simulink model "Fuzzy_Logic_MPPT_for_SolarPV"  (R2023b)
settings: Solver=ode45  StartTime=0.0  StopTime=10  RelTol=1e-3  EnableMultiTasking=on
PostLoadFcn:
  | fuzzyLogicDesigner('mppt')
libraries: spsSeriesRLCBranchLib x4, spsDiodeLib x2, fuzblock x1, spsPWMGeneratorDCDCLib x1, spsMosfetLib x1, spsPVArrayLib x1, spsVoltageMeasurementLib x1, sps_lib x1
settings Model: Creator=Niaz  LastModifiedBy=SUCHINTH
settings SolverCC: AlgebraicLoopSolver=TrustRegion
settings DataIOCC: LimitDataPoints=on  SaveFormat=Array  ReturnWorkspaceOutputs=off
settings OptimizationCC: LifeSpan=inf
settings DebuggingCC: UnconnectedInputMsg=warning  UnconnectedOutputMsg=warning  UnconnectedLineMsg=warning  SFUnexpectedBacktrackingDiag=warning  SFNoUnconditionalDefaultTransitionDiag=warning  SFExecutionAtInitializationDiag=none  ArithmeticOperatorsInVariantConditions=warning
settings HardwareCC: ProdBitPerPointer=32  ProdBitPerSizeT=32  ProdBitPerPtrDiffT=32  ProdLargestAtomicFloat=None  ProdIntDivRoundTo=Undefined  ProdEndianess=Unspecified  ProdWordSize=32  ProdHWDeviceType=32-bit Generic
settings ModelReferenceCC: EnableRefExpFcnMdlSchedulingChecks=on  PropagateSignalLabelsOutOfModel=off
settings SFSimCC: SimUseLocalCustomCode=off  CustomCodeUndefinedFunction=UseInterfaceOnly
settings RTWCC: RTWUseLocalCustomCode=off
settings CodeAppCC: StateflowObjectComments=on
settings GRTTargetCC: TargetLangStandard=C89/C90 (ANSI)
settings ConfigComp: CovMetricSettings=dw  CovSaveCumulativeToWorkspaceVar=on  CovSaveSingleToWorkspaceVar=on  CovExternalEMLEnable=off
settings SimscapeCC: SimscapeNormalizeSystem=off  SimscapeLogType=all  SimscapeLogSimulationStatistics=on  SimscapeLogOpenViewer=on

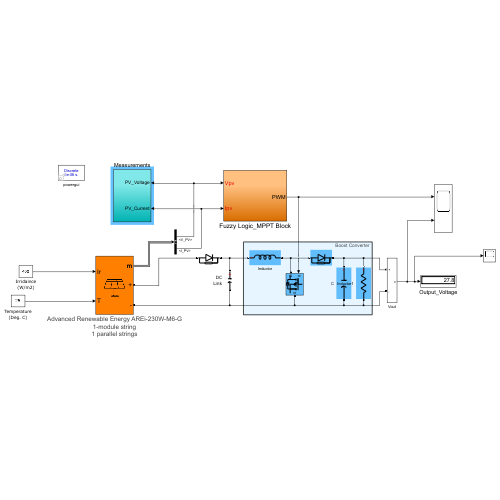
[thumbnail: Simulink's stored preview of the top-level diagram]
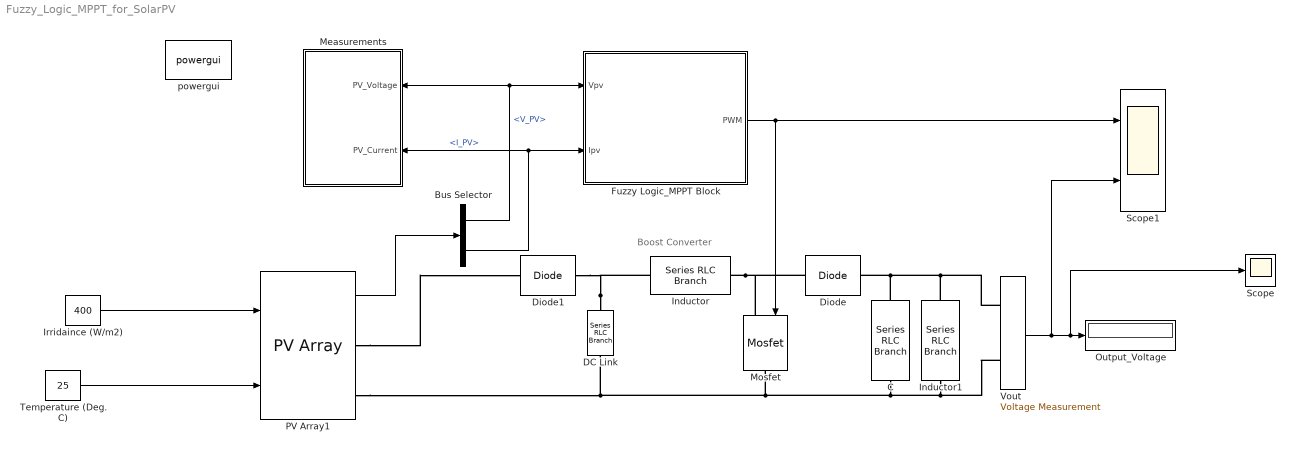
== system Fuzzy_Logic_MPPT_for_SolarPV ==
  note: Boost Converter
  Bus Selector : BusSelector  OutputSignals=V_PV,I_PV
  C : spsSeriesRLCBranchLib/Series RLC Branch  LConnTagsString=__new0  RConnTagsString=__new0  BranchType=C  Resistance=1  Inductance=1e-3  SetiL0=off  InitialCurrent=0  Capacitance=5000e-6  Setx0=off  InitialVoltage=600  Measurements=None
  DC Link : spsSeriesRLCBranchLib/Series RLC Branch  LConnTagsString=__new0  RConnTagsString=__new0  BranchType=C  Resistance=0.001  Inductance=1.0  SetiL0=off  InitialCurrent=0  Capacitance=4000e-6  Setx0=off  InitialVoltage=310  Measurements=None
  Diode : spsDiodeLib/Diode  Ron=0.001  Lon=0  Vf=0.8  IC=0  UseSnubber=off  Rs=500  Cs=250e-9  Measurements=off
  Diode1 : spsDiodeLib/Diode  Ron=0.001  Lon=0  Vf=0.8  IC=0  UseSnubber=off  Rs=500  Cs=250e-9  Measurements=off
  Fuzzy Logic_MPPT Block : Subsystem
  Inductor : spsSeriesRLCBranchLib/Series RLC Branch  LConnTagsString=__new0  RConnTagsString=__new0  BranchType=L  Resistance=0.01  Inductance=4e-4  SetiL0=off  InitialCurrent=5  Capacitance=1e-6  Setx0=off  InitialVoltage=0  Measurements=None
  Inductor1 : spsSeriesRLCBranchLib/Series RLC Branch  LConnTagsString=__new0  RConnTagsString=__new0  BranchType=R  Resistance=10  Inductance=4e-4  SetiL0=off  InitialCurrent=5  Capacitance=1e-6  Setx0=off  InitialVoltage=0  Measurements=None
  Irridaince (W/m2) : Constant  Value=400
  Measurements : Subsystem
  Mosfet : spsMosfetLib/Mosfet  Ron=0.1  Lon=0  Rd=0.01  Vfd=0  IC=0  Rs=1e5  Cs=inf  Measurements=off
  Output_Voltage : Display
  PV Array1 : spsPVArrayLib/PV Array  Npar=1  Nser=1  PlotType=one module @ 25 deg.C & specified irradiances  S_vec=[1000 800 400 200 100]  Temp_C_vec=[ 50 ]  ModuleName=Advanced Renewable Energy AREi-230W-M6-G  PlotWhenSelected=off  Pm=230.4  Ncell=60  Voc=37.14  Isc=8  Vm=30.72  Im=7.5  beta_Voc_pc=-0.35335  alpha_Isc_pc=0.05535  beta_Voc=-0.13123  alpha_Isc=0.004428  IL=8.007  I0=2.1265e-10  nI=0.99005  Rsh=280.3446  Rs=0.2449  RobustModel=off  RobustCellTemperature=313.3991  BAL=on  Tc=1e-6  Tfilter=5e-5
      settings: AttributesFormatString=|
      | %<ModuleName>
      | %<Nser>-module string
      | %<Npar> parallel strings
  Scope : Scope
  Scope1 : Scope  NumInputPorts=2
  Temperature (Deg. C) : Constant  Value=25
  Vout : spsVoltageMeasurementLib/Voltage Measurement  PhasorSimulation=off  OutputType=Complex  PSBequivalent=0
  powergui : sps_lib/powergui  Priority=1  SimulationMode=Discrete  SampleTime=5e-6  frequency=60  Iterations=50  frequencyindice=0  Pbase=100e6  ErrMax=1e-4  UnitsV=kV  UnitsW=MW  buscounter=0  FunctionMessages=off  echomessages=off  EnableUseOfTLC=off  CurrentSourceSwitches=off  DisableSnubberDevices=off  DisableRonSwitches=off  DisableVfSwitches=off  DisplayEquations=off  AutomaticDiscreteSolvers=off  SolverType=Tustin/Backward Euler (TBE)  Interpol=off  ExternalGateDelay=off  methode=off  Ts=100  x0status=blocks  SPID=off  SwTol=0  HookPort=off  NonlinearTolerance=1e-4  nMaxIteration=100  ContinueOnMaxIteration=off  RestoreLinks=warning  ResistiveCurrentMeasurement=off  Frange=[0:2:500]  Ylog=off  Xlog=on  ShowGrid=off  save=off  variable=ZData  structure=0  ZoomFFT=off  StartTime=0.0  cycles=1  DisplayStyle=1  fundamental=60  FreqAxis=off  MaxFrequency=1000  frequencyindicesteady=1  RmsSteady=1  display=off
  wires:
  PV Array1/1 -> Bus Selector/1
  Vout/1 -> Scope1/2, Scope/1, Output_Voltage/1
  Temperature (Deg. C)/1 -> PV Array1/2
  Fuzzy Logic_MPPT Block/1(PWM) -> Mosfet/1, Scope1/1
  Bus Selector/1 -> Measurements/1(PV_Voltage), Fuzzy Logic_MPPT Block/1(Vpv)  "<V_PV>"
  Bus Selector/2 -> Measurements/2(PV_Current), Fuzzy Logic_MPPT Block/2(Ipv)  "<I_PV>"
  Irridaince (W/m2)/1 -> PV Array1/1
  connections:
  DC Link/LConn1 -- Inductor/LConn1 -- Diode1/RConn1
  Vout/LConn2 -- Inductor1/RConn1 -- C/RConn1 -- Mosfet/RConn1 -- PV Array1/RConn2 -- DC Link/RConn1
  Vout/LConn1 -- Inductor1/LConn1 -- Diode/RConn1 -- C/LConn1
  Inductor/RConn1 -- Diode/LConn1 -- Mosfet/LConn1
  PV Array1/RConn1 -- Diode1/LConn1

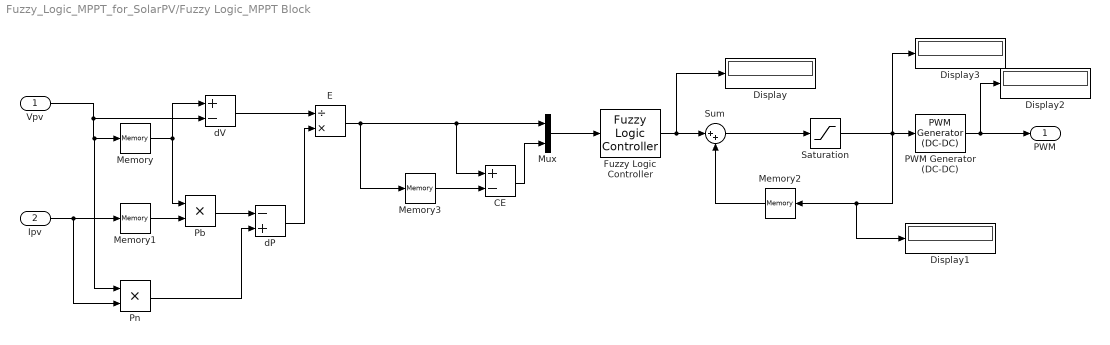
== system Fuzzy_Logic_MPPT_for_SolarPV/Fuzzy Logic_MPPT Block ==
  Vpv : Inport
  Ipv : Inport  Port=2
  CE : Sum  Inputs=+-
  Display{,1..3} (4 alike) : Display
  E : Product  Inputs=/*
  Fuzzy Logic Controller : fuzblock/Fuzzy Logic  Controller  FIS='fuzzy_mppt.fis'  OutputSampleNumber=101  DataType=double  FuzzifiedInputs=off  RuleFiringStrengths=off  RuleOutputs=off  AggregatedOutputs=off  SimulateUsing=Interpreted execution  OutOfRangeInputValueMessage=warning  NoRuleFiredMessage=warning  EmptyOutputFuzzySetMessage=warning
  Memory{,1..3} (4 alike) : Memory  InheritSampleTime=on
  Mux : Mux  Inputs=2
  PWM Generator (DC-DC) : spsPWMGeneratorDCDCLib/PWM Generator (DC-DC)  Fsw=10000  Ts=0
  Pb : Product
  Pn : Product
  Saturation : Saturate  UpperLimit=0.9  LowerLimit=0.1
  Sum : Sum  Inputs=|++
  dP : Sum  Inputs=-+
  dV : Sum  Inputs=+-
  PWM : Outport  VectorParamsAs1DForOutWhenUnconnected=off
  wires:
  Memory/1 -> dV/1, Pb/1
  Ipv/1 -> Pn/2, Memory1/1
  Memory1/1 -> Pb/2
  Pb/1 -> dP/1
  Pn/1 -> dP/2
  Mux/1 -> Fuzzy Logic Controller/1
  Memory2/1 -> Sum/2
  Memory3/1 -> CE/2
  CE/1 -> Mux/2
  PWM Generator (DC-DC)/1 -> Display2/1, PWM/1
  Vpv/1 -> dV/2, Pn/1, Memory/1
  dP/1 -> E/2
  E/1 -> Mux/1, CE/1, Memory3/1
  dV/1 -> E/1
  Saturation/1 -> Display1/1, Memory2/1, Display3/1, PWM Generator (DC-DC)/1
  Fuzzy Logic Controller/1 -> Display/1, Sum/1
  Sum/1 -> Saturation/1

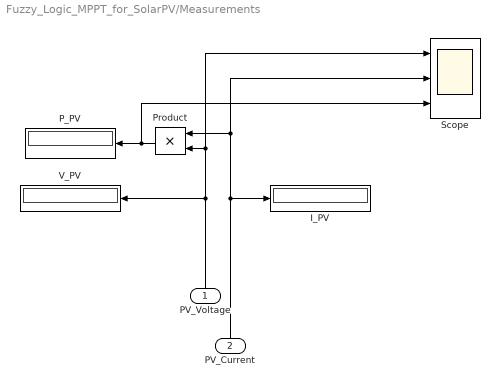
== system Fuzzy_Logic_MPPT_for_SolarPV/Measurements ==
  PV_Voltage : Inport
  PV_Current : Inport  Port=2
  I_PV : Display
  P_PV : Display
  Product : Product
  Scope : Scope  NumInputPorts=3
  V_PV : Display
  wires:
  Product/1 -> Scope/3, P_PV/1
  PV_Current/1 -> Product/1, Scope/2, I_PV/1
  PV_Voltage/1 -> Product/2, Scope/1, V_PV/1
